simulink model "one"  (R2014a)
settings: Solver=ode45  StartTime=0.0  StopTime=10.0  MaxStep=0.001  MinStep=0.00001  RelTol=1e-3
settings Model: Creator=trigg  LastModifiedBy=trigg

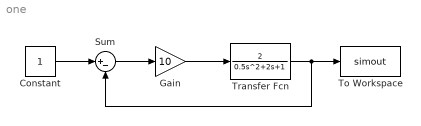
== system one ==
  Constant : Constant
  Gain : Gain  Gain=10
  Sum : Sum  Inputs=|+-
  To Workspace : ToWorkspace  VariableName=simout  SaveFormat=Timeseries  SampleTime=-1
  Transfer Fcn : TransferFcn  Numerator=[2]  Denominator=[0.5 2 1]
  wires:
  Constant/1 -> Sum/1
  Sum/1 -> Gain/1
  Gain/1 -> Transfer Fcn/1
  Transfer Fcn/1 -> To Workspace/1, Sum/2
